simulink model "InteractiveArmModel_R2021a_v1"  (R2021a)
settings: Solver=ode4  StartTime=0.0  StopTime=3000  FixedStep=1/150  MaxStep=1/50  MinStep=1/200  RelTol=1e-5  AbsTol=1e-6  EnableMultiTasking=on
model workspace (MAT data in the model file):
  MaxEccentricFlexor = 0.5
  PoleZ = 0.85
  SampleTime = 0.05
  musNoise = 0
  musNoiseLevel = Simulink.Parameter
  musNoiseLevel.Value = 15.23
  musNoiseLevel.DataType = 'auto'
  musNoiseLevel.Dimensions = [1 1]
libraries: simulink x1
(part 1 of 3)
Description:
  | An interactive musculoskeletal model controllable with electromyography.
settings Model: SILPILModeSetting=veronly  PacingRate=1000  ExtModeTrigDuration=2  VariantFading=off  OrderedModelArguments=off  Creator=Christopher J. Hasson  LastModifiedBy=cjhas
settings SolverCC: AutoScaleAbsTol=off  InitialStep=1/10  ZeroCrossAlgorithm=Adaptive  AlgebraicLoopSolver=TrustRegion
settings OptimizationCC: DefaultParameterBehavior=Inlined  EnhancedBackFolding=on  PassReuseOutputArgsAs=Individual arguments  ZeroExternalMemoryAtStartup=off  ZeroInternalMemoryAtStartup=off  MaxStackSize=64  OptimizeBlockOrder=speed  DifferentSizesBufferReuse=on  OptimizationCustomize=off  EfficientTunableParamExpr=on
settings DebuggingCC: ReadBeforeWriteMsg=DisableAll  WriteAfterWriteMsg=DisableAll  WriteAfterReadMsg=DisableAll  MultiTaskDSMMsg=none  ParameterTunabilityLossMsg=error  SFMachineParentedDataDiag=warning
settings HardwareCC: ProdBitPerInt=16  ProdBitPerPointer=16  ProdBitPerSizeT=16  ProdBitPerPtrDiffT=16  ProdLargestAtomicFloat=None  ProdWordSize=8  ProdHWDeviceType=Atmel->AVR  UseEmbeddedCoderFeatures=off
settings ModelReferenceCC: UpdateModelReferenceTargets=IfOutOfDate
settings SFSimCC: SFSimEcho=off  MATLABDynamicMemAlloc=off
settings RTWCC: SystemTargetFile=ert.tlc  TemplateMakefile=ert_default_tmf  Toolchain=Arduino AVR  BuildConfiguration=Faster Runs
settings CodeAppCC: ForceParamTrailComments=on  IgnoreCustomStorageClasses=off  OperatorAnnotations=on  SimulinkDataObjDesc=on  SFDataObjDesc=on  InsertBlockDesc=on
settings ERTTargetCC: SupportContinuousTime=on  SupportNonInlinedSFcns=on  SupportVariableSizeSignals=on  ExtModeStaticAllocSize=250  ERTCustomFileTemplate=example_file_process.tlc

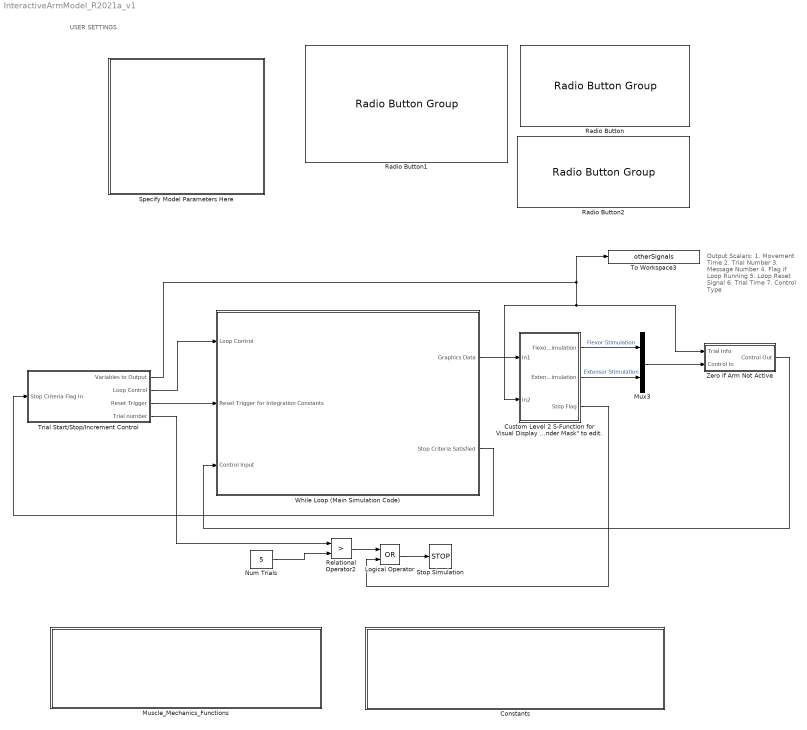
== system InteractiveArmModel_R2021a_v1 ==
  note: Output Scalars:
      | 1. Movement Time
      | 2. Trial Number
      | 3. Message Number
      | 4. Flag if Loop Running
      | 5. Loop Reset Signal
      | 6. Trial Time
      | 7. Control Type
  note: USER SETTINGS
  Constants : Subsystem
  "Custom Level 2 S-Function for Visual Display and Controls [Calls \"InteractiveDisplay.m\"] Select \"Look Under Mask\" to edit." : Subsystem  mask(Mutiple XY Graph){number_of_trajectories=2, axis_limits=[-0.5 0.5 -0.5 0.5], sample_time=0.01}
      mask prompts: number_of_trajectories "Number of Trajectories"; axis_limits "Axis Limits"; sample_time "Sample Time"
      mask Display: plot([.05 .95 .95 .05 .05],[.45 .45 .95 .95 .45], 0.5+cos(0:0.1:2*pi)*0.3,0.7+sin(0:0.1:2*pi)*0.2)
  Logical Operator : Logic  Operator=OR  AllPortsSameDT=off  OutDataTypeStr=boolean
  Muscle_Mechanics_Functions : Subsystem
  Mux3 : Mux  Inputs=2
  Num Trials : Constant  Value=5
  Radio Button : RadioButtonGroup  LabelPosition=Hide  SelectedLabel=Keyboard  ButtonGroupName=Control Mode
      settings: Values={{'Keyboard', 'Mouse', 'EMG'}, [0 1 2]}
  Radio Button1 : RadioButtonGroup  LabelPosition=Hide  SelectedLabel=Muscle Model  ButtonGroupName=Actuation
      settings: Values={{'Muscle Model', 'Force Generator', 'Torque Generator'}, [0 1 2]}
  Radio Button2 : RadioButtonGroup  LabelPosition=Hide  SelectedLabel=Normal  ButtonGroupName=Model Muscle Strength
      settings: Values={{'Normal', 'Weak (50% Reduction)'}, [0 1]}
  Relational Operator2 : RelationalOperator  Operator=>  RndMeth=Simplest
  Specify Model Parameters Here : Subsystem
  Stop Simulation : Stop
  To Workspace3 : ToWorkspace  VariableName=otherSignals  SaveFormat=Timeseries  SampleTime=-1
  Trial Start/Stop/Increment Control : Subsystem
  While Loop (Main Simulation Code) : Subsystem  TreatAsAtomicUnit=on
  Zero if Arm Not Active : Subsystem
  wires:
  While Loop (Main Simulation Code)/1(Graphics Data) -> "Custom Level 2 S-Function for Visual Display and Controls [Calls \"InteractiveDisplay.m\"] Select \"Look Under Mask\" to edit."/1(In1)
  Mux3/1 -> Zero if Arm Not Active/2(Control In)
  Zero if Arm Not Active/1(Control Out) -> While Loop (Main Simulation Code)/3(Control Input)
  "Custom Level 2 S-Function for Visual Display and Controls [Calls \"InteractiveDisplay.m\"] Select \"Look Under Mask\" to edit."/1(Flexor Stimulation) -> Mux3/1  "Flexor Stimulation"
  "Custom Level 2 S-Function for Visual Display and Controls [Calls \"InteractiveDisplay.m\"] Select \"Look Under Mask\" to edit."/2(Extensor Stimulation) -> Mux3/2  "Extensor Stimulation"
  Num Trials/1 -> Relational Operator2/2
  Relational Operator2/1 -> Logical Operator/1
  "Custom Level 2 S-Function for Visual Display and Controls [Calls \"InteractiveDisplay.m\"] Select \"Look Under Mask\" to edit."/3(Stop Flag) -> Logical Operator/2
  Logical Operator/1 -> Stop Simulation/1
  Trial Start/Stop/Increment Control/1(Variables to Output) -> Zero if Arm Not Active/1(Trial Info), "Custom Level 2 S-Function for Visual Display and Controls [Calls \"InteractiveDisplay.m\"] Select \"Look Under Mask\" to edit."/2(In2), To Workspace3/1
  While Loop (Main Simulation Code)/2(Stop Criteria Satisfied) -> Trial Start/Stop/Increment Control/1(Stop Criteria Flag In)
  Trial Start/Stop/Increment Control/4(Trial number) -> Relational Operator2/1
  Trial Start/Stop/Increment Control/2(Loop Control) -> While Loop (Main Simulation Code)/1(Loop Control)
  Trial Start/Stop/Increment Control/3(Reset Trigger) -> While Loop (Main Simulation Code)/2(Reset Trigger for Integration Constants)

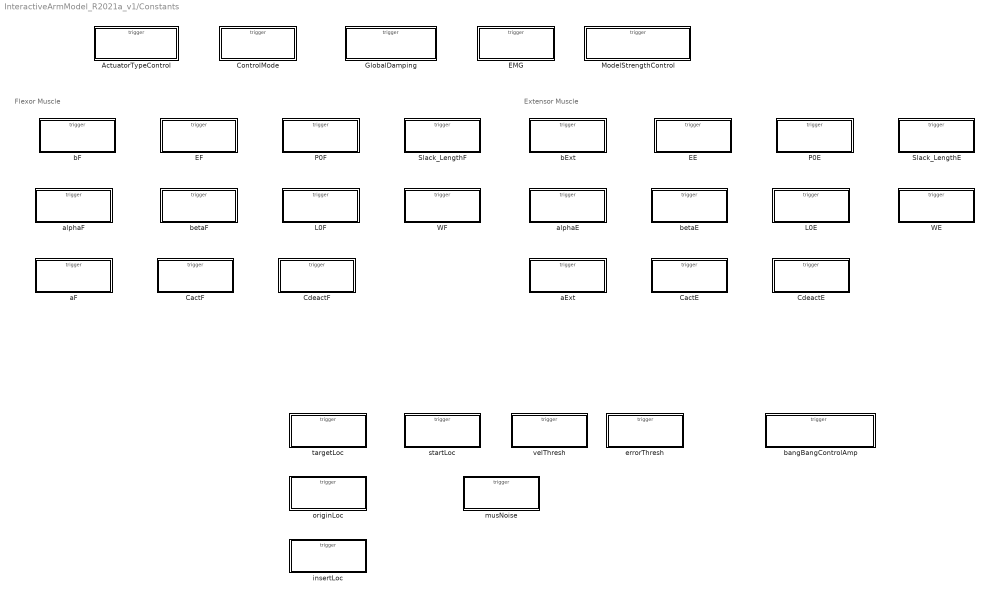
== system InteractiveArmModel_R2021a_v1/Constants ==
  note: Extensor Muscle
  note: Flexor Muscle
  ActuatorTypeControl : Subsystem  TreatAsAtomicUnit=on
  CactE : Subsystem  TreatAsAtomicUnit=on
  CactF : Subsystem  TreatAsAtomicUnit=on
  CdeactE : Subsystem  TreatAsAtomicUnit=on
  CdeactF : Subsystem  TreatAsAtomicUnit=on
  ControlMode : Subsystem  TreatAsAtomicUnit=on
  EE : Subsystem  TreatAsAtomicUnit=on
  EF : Subsystem  TreatAsAtomicUnit=on
  EMG : Subsystem  TreatAsAtomicUnit=on
  GlobalDamping : Subsystem  TreatAsAtomicUnit=on
  L0E : Subsystem  TreatAsAtomicUnit=on
  L0F : Subsystem  TreatAsAtomicUnit=on
  ModelStrengthControl : Subsystem  TreatAsAtomicUnit=on
  P0E : Subsystem  TreatAsAtomicUnit=on
  P0F : Subsystem  TreatAsAtomicUnit=on
  Slack_LengthE : Subsystem  TreatAsAtomicUnit=on
  Slack_LengthF : Subsystem  TreatAsAtomicUnit=on
  WE : Subsystem  TreatAsAtomicUnit=on
  WF : Subsystem  TreatAsAtomicUnit=on
  aExt : Subsystem  TreatAsAtomicUnit=on
  aF : Subsystem  TreatAsAtomicUnit=on
  alphaE : Subsystem  TreatAsAtomicUnit=on
  alphaF : Subsystem  TreatAsAtomicUnit=on
  bExt : Subsystem  TreatAsAtomicUnit=on
  bF : Subsystem  TreatAsAtomicUnit=on
  bangBangControlAmp : Subsystem  TreatAsAtomicUnit=on
  betaE : Subsystem  TreatAsAtomicUnit=on
  betaF : Subsystem  TreatAsAtomicUnit=on
  errorThresh : Subsystem  TreatAsAtomicUnit=on
  insertLoc : Subsystem  TreatAsAtomicUnit=on
  musNoise : Subsystem  TreatAsAtomicUnit=on
  originLoc : Subsystem  TreatAsAtomicUnit=on
  startLoc : Subsystem  TreatAsAtomicUnit=on
  targetLoc : Subsystem  TreatAsAtomicUnit=on
  velThresh : Subsystem  TreatAsAtomicUnit=on

== system InteractiveArmModel_R2021a_v1/Custom Level 2 S-Function for Visual Display and Controls [Calls "InteractiveDisplay.m"] Select "Look Under Mask" to edit. ==
  In1 : Inport
  In2 : Inport  Port=2
  Demux : Demux  Outputs=25
  Level-2 MATLAB S-Function : M-S-Function  FunctionName=InteractiveDisplay  Parameters=number_of_trajectories,axis_limits
  Flexor Stimulation : Outport
  Extensor Stimulation : Outport  Port=2
  Stop Flag : Outport  Port=3
  wires:
  Level-2 MATLAB S-Function/1 -> Demux/1
  Demux/1 -> Flexor Stimulation/1
  Demux/2 -> Extensor Stimulation/1
  In1/1 -> Level-2 MATLAB S-Function/1
  In2/1 -> Level-2 MATLAB S-Function/2
  Demux/3 -> Stop Flag/1

== system InteractiveArmModel_R2021a_v1/Muscle_Mechanics_Functions ==
  Contractile Element Excitation-Activation Relation : Subsystem  TreatAsAtomicUnit=on
  Contractile Element Force-Length Relation : Subsystem  TreatAsAtomicUnit=on
  Contractile Element Force-Velocity Relation : Subsystem  TreatAsAtomicUnit=on
  "Series-Elastic Element Stiffness Relation " : Subsystem  TreatAsAtomicUnit=on

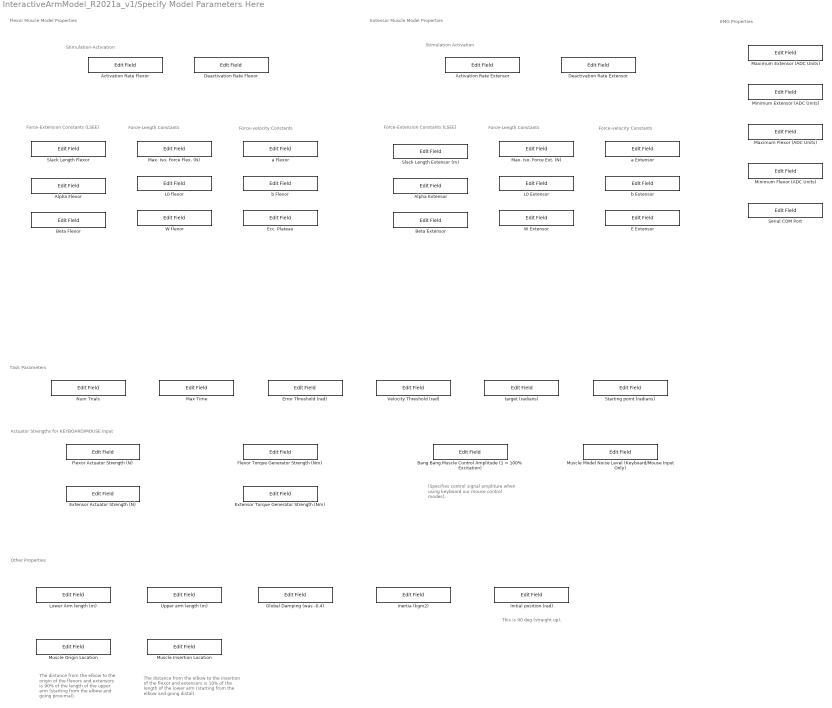
== system InteractiveArmModel_R2021a_v1/Specify Model Parameters Here ==
  note: (Specifies control signal ampliture when using keyboard our mouse control modes).
  note: EMG Properties
  note: Task Parameters
  note: Stimulation Activation
  note: Stimulation-Activation
  note: Force-velocity Constants
  note: Force-Extension Constants
      |  (LSEE)
  note: Force-Length Constants
  note: Flexor Muscle Model Properties
  note: Extensor Muscle Model Properties
  note: Force-velocity Constants
  note: Force-Extension Constants
      |  (LSEE)
  note: Force-Length Constants
  note: Actuator Strengths for KEYBOARD/MOUSE Input
  note: The distance from the elbow to the origin of the flexors and extensors is 90% of the length of the upper arm (starting from the elbow and going proximal).
  note: The distance from the elbow to the insertion of the flexor and extensors is 10% of the length of the lower arm (starting from the elbow and going distal).
  note: This is 90 deg (straight up).
  note: Other Properties
  Activation Rate Extensor : EditField  LabelPosition=Hide  ShowInitialText=on  Alignment=Center
  Activation Rate Flexor : EditField  LabelPosition=Hide  ShowInitialText=on  Alignment=Center
  Alpha Extensor : EditField  LabelPosition=Hide  ShowInitialText=on  Alignment=Center
  Alpha Flexor : EditField  LabelPosition=Hide  ShowInitialText=on  Alignment=Center
  Bang Bang Muscle Control Amplitude (1 = 100% Excitation) : EditField  LabelPosition=Hide  ShowInitialText=on  Alignment=Center
  Beta Extensor : EditField  LabelPosition=Hide  ShowInitialText=on  Alignment=Center
  Beta Flexor : EditField  LabelPosition=Hide  ShowInitialText=on  Alignment=Center
  Deactivation Rate Extensor : EditField  LabelPosition=Hide  ShowInitialText=on  Alignment=Center
  Deactivation Rate Flexor : EditField  LabelPosition=Hide  ShowInitialText=on  Alignment=Center
  E Extensor : EditField  LabelPosition=Hide  ShowInitialText=on  Alignment=Center
  Ecc. Plateau : EditField  LabelPosition=Hide  ShowInitialText=on  Alignment=Center
  Error Threshold (rad) : EditField  LabelPosition=Hide  ShowInitialText=on  Alignment=Center
  Extensor Actuator Strength (N) : EditField  LabelPosition=Hide  ShowInitialText=on  Alignment=Center
  Extensor Torque Generator Strength (Nm) : EditField  LabelPosition=Hide  ShowInitialText=on  Alignment=Center
  Flexor Actuator Strength (N) : EditField  LabelPosition=Hide  ShowInitialText=on  Alignment=Center
  Flexor Torque Generator Strength (Nm) : EditField  LabelPosition=Hide  ShowInitialText=on  Alignment=Center
  Global Damping (was -0.4) : EditField  LabelPosition=Hide  ShowInitialText=on  Alignment=Center
  Inertia (kgm2) : EditField  LabelPosition=Hide  ShowInitialText=on  Alignment=Center
  Initial position (rad) : EditField  LabelPosition=Hide  ShowInitialText=on  Alignment=Center
  L0 Extensor : EditField  LabelPosition=Hide  ShowInitialText=on  Alignment=Center
  L0 flexor : EditField  LabelPosition=Hide  ShowInitialText=on  Alignment=Center
  Lower Arm length (m) : EditField  LabelPosition=Hide  ShowInitialText=on  Alignment=Center
  Max Time : EditField  LabelPosition=Hide  ShowInitialText=on  Alignment=Center
  Max. Iso. Force Ext. (N) : EditField  LabelPosition=Hide  ShowInitialText=on  Alignment=Center
  Max. Iso. Force Flex. (N) : EditField  LabelPosition=Hide  ShowInitialText=on  Alignment=Center
  Maximum Extensor (ADC Units) : EditField  LabelPosition=Hide  ShowInitialText=on  Alignment=Center
  Maximum Flexor (ADC Units) : EditField  LabelPosition=Hide  ShowInitialText=on  Alignment=Center
  Minimum Extensor (ADC Units) : EditField  LabelPosition=Hide  ShowInitialText=on  Alignment=Center
  Minimum Flexor (ADC Units) : EditField  LabelPosition=Hide  ShowInitialText=on  Alignment=Center
  Muscle Insertion Location : EditField  LabelPosition=Hide  ShowInitialText=on  Alignment=Center
  Muscle Model Noise Level (Keyboard/Mouse Input Only) : EditField  LabelPosition=Hide  ShowInitialText=on  Alignment=Center
  Muscle Origin Location : EditField  LabelPosition=Hide  ShowInitialText=on  Alignment=Center
  Num Trials : EditField  LabelPosition=Hide  ShowInitialText=on  Alignment=Center
  Serial COM Port : EditField  LabelPosition=Hide  ShowInitialText=on  Alignment=Center
  Slack Length Extensor (m) : EditField  LabelPosition=Hide  ShowInitialText=on  Alignment=Center
  Slack Length Flexor : EditField  LabelPosition=Hide  ShowInitialText=on  Alignment=Center
  Starting point (radians) : EditField  LabelPosition=Hide  ShowInitialText=on  Alignment=Center
  Upper arm length (m) : EditField  LabelPosition=Hide  ShowInitialText=on  Alignment=Center
  Velocity Threshold (rad) : EditField  LabelPosition=Hide  ShowInitialText=on  Alignment=Center
  W Extensor : EditField  LabelPosition=Hide  ShowInitialText=on  Alignment=Center
  W flexor : EditField  LabelPosition=Hide  ShowInitialText=on  Alignment=Center
  a Extensor : EditField  LabelPosition=Hide  ShowInitialText=on  Alignment=Center
  a Flexor : EditField  LabelPosition=Hide  ShowInitialText=on  Alignment=Center
  b Extensor : EditField  LabelPosition=Hide  ShowInitialText=on  Alignment=Center
  b Flexor : EditField  LabelPosition=Hide  ShowInitialText=on  Alignment=Center
  target (radians) : EditField  LabelPosition=Hide  ShowInitialText=on  Alignment=Center

== system InteractiveArmModel_R2021a_v1/Trial Start//Stop//Increment Control ==
  note: 1 = Trial is active (Stop critiera not satisfied and trial time hasn't reached limit).
  Stop Criteria Flag In : Inport
  Counter for Trial Number : Subsystem  TreatAsAtomicUnit=on
  Data Type Conversion2 : DataTypeConversion
  Delay : Delay  DelayLength=50  InitialCondition=0
  Extract Movement Time : Subsystem  TreatAsAtomicUnit=on
  Flag for What Phase Trial is In : Subsystem
  Function Caller : FunctionCaller  FunctionPrototype=y = Constants.ControlMode()  OutputArgumentSpecifications=<Enter example>
  Mux : Mux  Inputs=7
  Reset Trigger Logic : Subsystem
  Stop Criteria Flag Control (Between Trials) : Subsystem
  Subsystem : Subsystem
  Subsystem1 : Subsystem
  Subsystem2 : Subsystem
  Variables to Output : Outport
  Loop Control : Outport  Port=2
  Reset Trigger : Outport  Port=3
  Trial number : Outport  Port=4
  wires:
  Subsystem2/1(IC) -> Loop Control/1, Extract Movement Time/Trigger, Mux/4
  Reset Trigger Logic/1(Reset Trigger) -> Reset Trigger/1, Data Type Conversion2/1
  Subsystem/1(Simulation Time) -> Subsystem2/1(Simulation Time)
  Subsystem1/2(Trial Time Flag) -> Flag for What Phase Trial is In/1(Trial Time Flag)
  Mux/1 -> Variables to Output/1
  Stop Criteria Flag Control (Between Trials)/1(Stop Criteria Flag Out) -> Subsystem1/2(Stop Criteria Flag), Flag for What Phase Trial is In/2(Stop Criteria Flag), Reset Trigger Logic/2(Stop Criteria Flag)
  Flag for What Phase Trial is In/1(message display) -> Mux/3
  Counter for Trial Number/1(Trial Number Switch) -> Trial number/1, Mux/2  "Trial number"
  Extract Movement Time/1(Movement Time) -> Mux/1
  Data Type Conversion2/1 -> Mux/5  "Reset"
  Subsystem/2(Trial Time) -> Counter for Trial Number/Trigger, Extract Movement Time/1(Trial Time), Mux/6, Reset Trigger Logic/1(Trial Time), Subsystem1/1(Trial Time)
  Function Caller/1 -> Mux/7
  Delay/1 -> Subsystem/1(In1)
  Subsystem1/1(StopCriteria&TrialTime Flag) -> Subsystem2/2(StopCriteria&TrialTime Flag), Delay/1
  Stop Criteria Flag In/1 -> Stop Criteria Flag Control (Between Trials)/1(Stop Criteria Flag In)

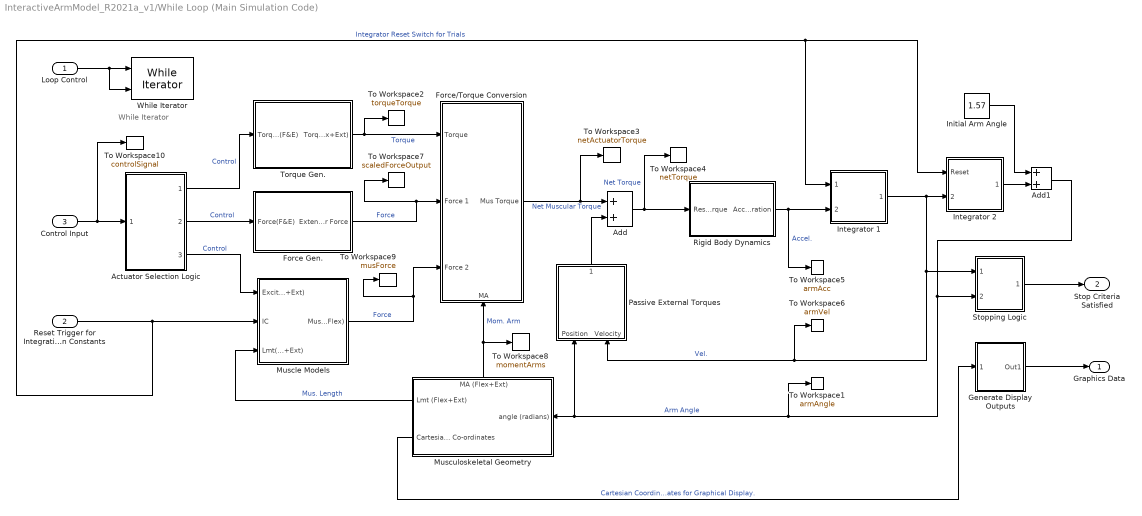
== system InteractiveArmModel_R2021a_v1/While Loop (Main Simulation Code) ==
  note: While Iterator
  Loop Control : Inport
  Reset Trigger for Integration Constants : Inport  Port=2
  Control Input : Inport  Port=3
  Actuator Selection Logic : Subsystem
  Add : Sum
  Add1 : Sum
  Force Gen. : Subsystem
  Force/Torque Conversion : Subsystem
      settings: PortSchema="{\"entries\":[{\"content\":{\"sides\":[{\"content\":{\"connectorIds\":[\"In1\",\"In2\",\"In3\"]},\"type\":\"ConnectorPlacement.EquallySpacedRectSide\",\"uuid\":\"3849f213-61a2-4952-aa4f-2be59b7e729a\"},{\"content\":{\"connectorIds\":[\"Out1\"],\"side\":\"RIGHT\"},\"type\":\"ConnectorPlacement.EquallySpacedRectSide\",\"uuid\":\"a03946d5-4adf-48f1-b5d4-befc99ec4479\"},{\"content\":{\"connectorIds\":[],\"side\":\"TOP\"},\"type\":\"ConnectorPlacement.EquallySpacedRectSide\",\"uuid\":\"26cd925e-d209-4c63-b11b-6b56fbf295e7\"},{\"content\":{\"connectorIds\":[\"In4\"],\"side\":\"BOTTOM\"},\"type\":\"ConnectorPlacement.EquallySpacedRectSide\",\"uuid\":\"3307b9fa-59bc-4d23-82dd-e0fccabeb078\"}]},\"type\":\"ConnectorPlacement.EquallySpacedConnector\",\"uuid\":\"629632a8-6ad9-402b-9008-6a2bdbad6252\"}],\"packageUris\":[\"http://schema.mathworks.com/mf0/Connector/R2020b\"],\"version\":\"1.0\"}"
  Generate Display Outputs : Subsystem
      settings: PortSchema="{\"entries\":[{\"content\":{\"sides\":[{\"content\":{\"connectorIds\":[\"Out1\"]},\"type\":\"ConnectorPlacement.EquallySpacedRectSide\",\"uuid\":\"907c53ba-e25a-48a3-8580-f053d35e8a8b\"},{\"content\":{\"connectorIds\":[\"In1\"],\"side\":\"RIGHT\"},\"type\":\"ConnectorPlacement.EquallySpacedRectSide\",\"uuid\":\"e6d73d20-9b05-462a-b014-b0e267ff725b\"},{\"content\":{\"connectorIds\":[],\"side\":\"TOP\"},\"type\":\"ConnectorPlacement.EquallySpacedRectSide\",\"uuid\":\"2f7da445-9925-4d1a-82a6-929fe983f70f\"},{\"content\":{\"connectorIds\":[],\"side\":\"BOTTOM\"},\"type\":\"ConnectorPlacement.EquallySpacedRectSide\",\"uuid\":\"a6d810bc-350c-475e-931f-1209d385d960\"}]},\"type\":\"ConnectorPlacement.EquallySpacedConnector\",\"uuid\":\"aaa2837d-0021-4fae-b2fd-c5fc5dc28df7\"}],\"packageUris\":[\"http://schema.mathworks.com/mf0/Connector/R2020b\"],\"version\":\"1.0\"}"
  Initial Arm Angle : Constant  Value=1.57
  Integrator 1 : Subsystem
  Integrator 2 : Subsystem
  Muscle Models : Subsystem
  Musculoskeletal Geometry : Subsystem
      settings: PortSchema="{\"entries\":[{\"content\":{\"sides\":[{\"content\":{\"connectorIds\":[]},\"type\":\"ConnectorPlacement.EquallySpacedRectSide\",\"uuid\":\"8c940fc8-64df-4196-ac14-c49096b27983\"},{\"content\":{\"connectorIds\":[\"Out1\"],\"side\":\"RIGHT\"},\"type\":\"ConnectorPlacement.EquallySpacedRectSide\",\"uuid\":\"009c2c09-14e0-422f-89fa-0830fe563124\"},{\"content\":{\"connectorIds\":[\"Out2\",\"Out3\"],\"side\":\"TOP\"},\"type\":\"ConnectorPlacement.EquallySpacedRectSide\",\"uuid\":\"84c5c2e7-ffda-4103-9912-3de94ad78eb8\"},{\"content\":{\"connectorIds\":[\"In1\"],\"side\":\"BOTTOM\"},\"type\":\"ConnectorPlacement.EquallySpacedRectSide\",\"uuid\":\"bc27ef22-e0e2-497d-b784-b185d27dfcbe\"}]},\"type\":\"ConnectorPlacement.EquallySpacedConnector\",\"uuid\":\"d3fcff10-aff8-4015-b565-4cd041df8c8d\"}],\"packageUris\":[\"http://schema.mathworks.com/mf0/Connector/19700101\"],\"version\":\"1.0\"}"
  Passive External Torques : Subsystem
      settings: PortSchema="{\"entries\":[{\"content\":{\"sides\":[{\"content\":{\"connectorIds\":[]},\"type\":\"ConnectorPlacement.EquallySpacedRectSide\",\"uuid\":\"d0cf707c-0e80-49c4-a718-ce527ee82e97\"},{\"content\":{\"connectorIds\":[],\"side\":\"RIGHT\"},\"type\":\"ConnectorPlacement.EquallySpacedRectSide\",\"uuid\":\"ee5fdd45-e6b2-4d3c-954e-bdf912ed2468\"},{\"content\":{\"connectorIds\":[\"Out1\"],\"side\":\"TOP\"},\"type\":\"ConnectorPlacement.EquallySpacedRectSide\",\"uuid\":\"54b9e406-3152-4f28-af7f-87d9f53bbd53\"},{\"content\":{\"connectorIds\":[\"In1\",\"In2\"],\"side\":\"BOTTOM\"},\"type\":\"ConnectorPlacement.EquallySpacedRectSide\",\"uuid\":\"aacaddaa-a99e-4423-a15d-1a454195a54f\"}]},\"type\":\"ConnectorPlacement.EquallySpacedConnector\",\"uuid\":\"bf7677b5-f77f-4845-ae2c-48e3ea7a2b50\"}],\"packageUris\":[\"http://schema.mathworks.com/mf0/Connector/19700101\"],\"version\":\"1.0\"}"
  Rigid Body Dynamics : Subsystem
  Stopping Logic : Subsystem
  To Workspace1 : ToWorkspace  VariableName=armAngle  SaveFormat=Timeseries  SampleTime=-1
  To Workspace10 : ToWorkspace  VariableName=controlSignal  SaveFormat=Timeseries  SampleTime=-1
  To Workspace2 : ToWorkspace  VariableName=torqueTorque  SaveFormat=Timeseries  SampleTime=-1
  To Workspace3 : ToWorkspace  VariableName=netActuatorTorque  SaveFormat=Timeseries  SampleTime=-1
  To Workspace4 : ToWorkspace  VariableName=netTorque  SaveFormat=Timeseries  SampleTime=-1
  To Workspace5 : ToWorkspace  VariableName=armAcc  SaveFormat=Timeseries  SampleTime=-1
  To Workspace6 : ToWorkspace  VariableName=armVel  SaveFormat=Timeseries  SampleTime=-1
  To Workspace7 : ToWorkspace  VariableName=scaledForceOutput  SampleTime=-1
  To Workspace8 : ToWorkspace  VariableName=momentArms  SaveFormat=Timeseries  SampleTime=-1
  To Workspace9 : ToWorkspace  VariableName=musForce  SampleTime=-1
  Torque Gen. : Subsystem
  While Iterator : WhileIterator  MaxIters=1  OutputDataType=double
  Graphics Data : Outport
  Stop Criteria Satisfied : Outport  Port=2
  wires:
  Loop Control/1 -> While Iterator/2, While Iterator/1
  Force/Torque Conversion/1(Mus Torque) -> To Workspace3/1, Add/1  "Net Muscular Torque"
  Passive External Torques/1(Net External Torque) -> Add/2
  Add/1 -> To Workspace4/1, Rigid Body Dynamics/1(Resultant torque)  "Net Torque"
  Muscle Models/1(Muscle Force (Ext+Flex)) -> To Workspace9/1, Force/Torque Conversion/3(Force 2)  "Force"
  Force Gen./1(Extensor Force) -> To Workspace7/1, Force/Torque Conversion/2(Force 1)  "Force"
  Musculoskeletal Geometry/1(MA (Flex+Ext)) -> Force/Torque Conversion/4(MA), To Workspace8/1  "Mom. Arm"
  Musculoskeletal Geometry/2(Cartesian Co-ordinates) -> Generate Display Outputs/1(Cartesian Co-ordinates)  "Cartesian Coordinates for Graphical Display."
  Add1/1 -> To Workspace1/1, Musculoskeletal Geometry/1(angle (radians)), Passive External Torques/1(Position), Stopping Logic/2(Angle (radians))  "Arm Angle"
  Musculoskeletal Geometry/3(Lmt (Flex+Ext)) -> Muscle Models/3(Lmt(flex+Ext))  "Mus. Length"
  Torque Gen./1(Torque (flex+Ext)) -> To Workspace2/1, Force/Torque Conversion/1(Torque)  "Torque"
  Generate Display Outputs/1(Out1) -> Graphics Data/1
  Reset Trigger for Integration Constants/1 -> Muscle Models/2(IC), Integrator 2/1(Reset), Integrator 1/1(Reset1)  "Integrator Reset Switch for Trials"
  Rigid Body Dynamics/1(" Acceleration") -> Integrator 1/2(Arm Accel.), To Workspace5/1  "Accel."
  Stopping Logic/1(Out2) -> Stop Criteria Satisfied/1
  Control Input/1 -> To Workspace10/1, Actuator Selection Logic/1(Control Input)
  Actuator Selection Logic/1(Torque Control Signal) -> Torque Gen./1(Torque(F&E))  "Control"
  Actuator Selection Logic/2(Force Actuator Control Signal) -> Force Gen./1(Force(F&E))  "Control"
  Integrator 1/1(Arm Vel.) -> To Workspace6/1, Passive External Torques/2(Velocity), Stopping Logic/1(Velocity (rad/s)), Integrator 2/2(Arm Vel.)  "Vel."
  Integrator 2/1(PosOut) -> Add1/2
  Initial Arm Angle/1 -> Add1/1
  Actuator Selection Logic/3(MuscleControlSignal) -> Muscle Models/1(Excitation(flex+Ext))  "Control"

== system InteractiveArmModel_R2021a_v1/Zero if Arm Not Active ==
  Trial Info : Inport
  Control In : Inport  Port=2
  Constant1 : Constant  Value=0
  Constant3 : Constant  Value=0
  Demux : Demux  Outputs=2
  Demux1 : Demux  Outputs=7
  If Action Subsystem1 : Subsystem  TreatAsAtomicUnit=on
  If Action Subsystem10 : Subsystem  TreatAsAtomicUnit=on
  If Action Subsystem11 : Subsystem  TreatAsAtomicUnit=on
  If Action Subsystem2 : Subsystem  TreatAsAtomicUnit=on
  If1 : If  IfExpression=u1 == 0
  If5 : If  IfExpression=u1 == 0
  Logical Operator : Logic  AllPortsSameDT=off  OutDataTypeStr=boolean
  Merge1 : Merge
  Merge4 : Merge
  Mux : Mux  Inputs=2
  Control Out : Outport
  wires:
  Constant3/1 -> If Action Subsystem10/1(In1)
  If Action Subsystem10/1(Out1) -> Merge4/1
  If5/1 -> If Action Subsystem10/Action
  If5/2 -> If Action Subsystem11/Action
  Merge4/1 -> Mux/1
  Mux/1 -> Control Out/1
  If Action Subsystem11/1(Out1) -> Merge4/2
  Constant1/1 -> If Action Subsystem1/1(In1)
  If1/1 -> If Action Subsystem1/Action
  Control In/1 -> Demux/1
  Demux/1 -> If Action Subsystem11/1(" ")  "Flexor"
  If1/2 -> If Action Subsystem2/Action
  Demux/2 -> If Action Subsystem2/1(" ")  "Extensor"
  If Action Subsystem2/1(Out1) -> Merge1/2
  If Action Subsystem1/1(Out1) -> Merge1/1
  Merge1/1 -> Mux/2
  Trial Info/1 -> Demux1/1
  Demux1/4 -> Logical Operator/1  "IC"
  Demux1/5 -> Logical Operator/2  "Reset"
  Logical Operator/1 -> If1/1, If5/1

== system InteractiveArmModel_R2021a_v1/Constants/ActuatorTypeControl ==
  ActuatorType : TriggerPort  TriggerType=function-call  IsSimulinkFunction=on  FunctionName=ActuatorType  FunctionVisibility=scoped  VariantControl=(inherit)
  Constant10 : Constant  Value=0
  y : ArgOut  DisableCoverage=on  ArgumentName=y
  wires:
  Constant10/1 -> y/1

== system InteractiveArmModel_R2021a_v1/Constants/CactE ==
  CactE : TriggerPort  TriggerType=function-call  IsSimulinkFunction=on  FunctionName=CactE  FunctionVisibility=scoped  VariantControl=(inherit)
  Flex Act Constant : Constant  Value=0.03
  y : ArgOut  DisableCoverage=on  ArgumentName=y
  wires:
  Flex Act Constant/1 -> y/1

== system InteractiveArmModel_R2021a_v1/Constants/CactF ==
  CactF : TriggerPort  TriggerType=function-call  IsSimulinkFunction=on  FunctionName=CactF  FunctionVisibility=scoped  VariantControl=(inherit)
  Flex Act Constant : Constant  Value=0.03
  y : ArgOut  DisableCoverage=on  ArgumentName=y
  wires:
  Flex Act Constant/1 -> y/1

== system InteractiveArmModel_R2021a_v1/Constants/CdeactE ==
  CdeactE : TriggerPort  TriggerType=function-call  IsSimulinkFunction=on  FunctionName=CdeactE  FunctionVisibility=scoped  VariantControl=(inherit)
  Ext Act Constant : Constant  Value=0.06
  y : ArgOut  DisableCoverage=on  ArgumentName=y
  wires:
  Ext Act Constant/1 -> y/1

== system InteractiveArmModel_R2021a_v1/Constants/CdeactF ==
  CdeactF : TriggerPort  TriggerType=function-call  IsSimulinkFunction=on  FunctionName=CdeactF  FunctionVisibility=scoped  VariantControl=(inherit)
  Flex Deact Constant : Constant  Value=0.06
  y : ArgOut  DisableCoverage=on  ArgumentName=y
  wires:
  Flex Deact Constant/1 -> y/1

== system InteractiveArmModel_R2021a_v1/Constants/ControlMode ==
  ControlMode : TriggerPort  TriggerType=function-call  IsSimulinkFunction=on  FunctionName=ControlMode  FunctionVisibility=scoped  VariantControl=(inherit)
  ControlModeConstant : Constant  Value=0
  y : ArgOut  DisableCoverage=on  ArgumentName=y
  wires:
  ControlModeConstant/1 -> y/1

== system InteractiveArmModel_R2021a_v1/Constants/EE ==
  EE : TriggerPort  TriggerType=function-call  IsSimulinkFunction=on  FunctionName=EE  FunctionVisibility=scoped  VariantControl=(inherit)
  eccentricExtensor : Constant  Value=3
  y : ArgOut  DisableCoverage=on  ArgumentName=y
  wires:
  eccentricExtensor/1 -> y/1

== system InteractiveArmModel_R2021a_v1/Constants/EF ==
  EF : TriggerPort  TriggerType=function-call  IsSimulinkFunction=on  FunctionName=EF  FunctionVisibility=scoped  VariantControl=(inherit)
  eccentricFlexor : Constant  Value=2.58
  y : ArgOut  DisableCoverage=on  ArgumentName=y
  wires:
  eccentricFlexor/1 -> y/1

== system InteractiveArmModel_R2021a_v1/Constants/EMG ==
  EMG : TriggerPort  TriggerType=function-call  IsSimulinkFunction=on  FunctionName=EMG  FunctionVisibility=scoped  VariantControl=(inherit)
  "EMG vs Button " : Constant  Value=0
  y : ArgOut  DisableCoverage=on  ArgumentName=y
  wires:
  "EMG vs Button "/1 -> y/1

== system InteractiveArmModel_R2021a_v1/Constants/GlobalDamping ==
  GlobalDamping : TriggerPort  TriggerType=function-call  IsSimulinkFunction=on  FunctionName=GlobalDamping  FunctionVisibility=scoped  VariantControl=(inherit)
  GlobalDampingConstant : Constant  Value=0
  y : ArgOut  DisableCoverage=on  ArgumentName=y
  wires:
  GlobalDampingConstant/1 -> y/1

== system InteractiveArmModel_R2021a_v1/Constants/L0E ==
  L0E : TriggerPort  TriggerType=function-call  IsSimulinkFunction=on  FunctionName=L0E  FunctionVisibility=scoped  VariantControl=(inherit)
  optLenExtensor : Constant  Value=0.223
  y : ArgOut  DisableCoverage=on  ArgumentName=y
  wires:
  optLenExtensor/1 -> y/1

== system InteractiveArmModel_R2021a_v1/Constants/L0F ==
  L0F : TriggerPort  TriggerType=function-call  IsSimulinkFunction=on  FunctionName=L0F  FunctionVisibility=scoped  VariantControl=(inherit)
  optLenFlex : Constant  Value=0.223
  y : ArgOut  DisableCoverage=on  ArgumentName=y
  wires:
  optLenFlex/1 -> y/1

== system InteractiveArmModel_R2021a_v1/Constants/ModelStrengthControl ==
  ModelStrengthControl : TriggerPort  TriggerType=function-call  IsSimulinkFunction=on  FunctionName=ModelStrengthControl  FunctionVisibility=scoped  VariantControl=(inherit)
  ModelStrengthConstant : Constant  Value=0
  y : ArgOut  DisableCoverage=on  ArgumentName=y
  wires:
  ModelStrengthConstant/1 -> y/1

== system InteractiveArmModel_R2021a_v1/Constants/P0E ==
  P0E : TriggerPort  TriggerType=function-call  IsSimulinkFunction=on  FunctionName=P0E  FunctionVisibility=scoped  VariantControl=(inherit)
  MaxIsoExtensor : Constant  Value=1000
  y : ArgOut  DisableCoverage=on  ArgumentName=y
  wires:
  MaxIsoExtensor/1 -> y/1

== system InteractiveArmModel_R2021a_v1/Constants/P0F ==
  P0F : TriggerPort  TriggerType=function-call  IsSimulinkFunction=on  FunctionName=P0F  FunctionVisibility=scoped  VariantControl=(inherit)
  MaxIsoFlexor : Constant  Value=1000
  y : ArgOut  DisableCoverage=on  ArgumentName=y
  wires:
  MaxIsoFlexor/1 -> y/1

== system InteractiveArmModel_R2021a_v1/Constants/Slack_LengthE ==
  Slack_lengthE : TriggerPort  TriggerType=function-call  IsSimulinkFunction=on  FunctionName=Slack_lengthE  FunctionVisibility=scoped  VariantControl=(inherit)
  SlackLenExt : Constant  Value=0.11
  y : ArgOut  DisableCoverage=on  ArgumentName=y
  wires:
  SlackLenExt/1 -> y/1

== system InteractiveArmModel_R2021a_v1/Constants/Slack_LengthF ==
  Slack_lengthF : TriggerPort  TriggerType=function-call  IsSimulinkFunction=on  FunctionName=Slack_lengthF  FunctionVisibility=scoped  VariantControl=(inherit)
  Slack_Length_Flexor : Constant  Value=0.12
  y : ArgOut  DisableCoverage=on  ArgumentName=y
  wires:
  Slack_Length_Flexor/1 -> y/1

== system InteractiveArmModel_R2021a_v1/Constants/WE ==
  WE : TriggerPort  TriggerType=function-call  IsSimulinkFunction=on  FunctionName=WE  FunctionVisibility=scoped  VariantControl=(inherit)
  widthExtensor : Constant  Value=0.036
  y : ArgOut  DisableCoverage=on  ArgumentName=y
  wires:
  widthExtensor/1 -> y/1

== system InteractiveArmModel_R2021a_v1/Constants/WF ==
  WF : TriggerPort  TriggerType=function-call  IsSimulinkFunction=on  FunctionName=WF  FunctionVisibility=scoped  VariantControl=(inherit)
  widthFlexor : Constant  Value=0.036
  y : ArgOut  DisableCoverage=on  ArgumentName=y
  wires:
  widthFlexor/1 -> y/1

== system InteractiveArmModel_R2021a_v1/Constants/aExt ==
  aE : TriggerPort  TriggerType=function-call  IsSimulinkFunction=on  FunctionName=aE  FunctionVisibility=scoped  VariantControl=(inherit)
  hillAExtensor : Constant  Value=360
  y : ArgOut  DisableCoverage=on  ArgumentName=y
  wires:
  hillAExtensor/1 -> y/1

== system InteractiveArmModel_R2021a_v1/Constants/aF ==
  aF : TriggerPort  TriggerType=function-call  IsSimulinkFunction=on  FunctionName=aF  FunctionVisibility=scoped  VariantControl=(inherit)
  hillAFlexor : Constant  Value=360
  y : ArgOut  DisableCoverage=on  ArgumentName=y
  wires:
  hillAFlexor/1 -> y/1

== system InteractiveArmModel_R2021a_v1/Constants/alphaE ==
  alphaE : TriggerPort  TriggerType=function-call  IsSimulinkFunction=on  FunctionName=alphaE  FunctionVisibility=scoped  VariantControl=(inherit)
  alphaExtensor : Constant  Value=605
  y : ArgOut  DisableCoverage=on  ArgumentName=y
  wires:
  alphaExtensor/1 -> y/1

== system InteractiveArmModel_R2021a_v1/Constants/alphaF ==
  alphaF : TriggerPort  TriggerType=function-call  IsSimulinkFunction=on  FunctionName=alphaF  FunctionVisibility=scoped  VariantControl=(inherit)
  alphaFlexor : Constant  Value=605
  y : ArgOut  DisableCoverage=on  ArgumentName=y
  wires:
  alphaFlexor/1 -> y/1

== system InteractiveArmModel_R2021a_v1/Constants/bExt ==
  bE : TriggerPort  TriggerType=function-call  IsSimulinkFunction=on  FunctionName=bE  FunctionVisibility=scoped  VariantControl=(inherit)
  hillBExtensor : Constant  Value=0.28
  y : ArgOut  DisableCoverage=on  ArgumentName=y
  wires:
  hillBExtensor/1 -> y/1

== system InteractiveArmModel_R2021a_v1/Constants/bF ==
  bF : TriggerPort  TriggerType=function-call  IsSimulinkFunction=on  FunctionName=bF  FunctionVisibility=scoped  VariantControl=(inherit)
  hillBFlexor : Constant  Value=0.28
  y : ArgOut  DisableCoverage=on  ArgumentName=y
  wires:
  hillBFlexor/1 -> y/1

== system InteractiveArmModel_R2021a_v1/Constants/bangBangControlAmp ==
  bangBangControlAmp : TriggerPort  TriggerType=function-call  IsSimulinkFunction=on  FunctionName=bangBangControlAmp  FunctionVisibility=scoped  VariantControl=(inherit)
  How Much Muscle Model is Activated using Keyboard/Mouse : Constant  Value=0.0349
  y : ArgOut  DisableCoverage=on  ArgumentName=y
  wires:
  How Much Muscle Model is Activated using Keyboard/Mouse/1 -> y/1

== system InteractiveArmModel_R2021a_v1/Constants/betaE ==
  betaE : TriggerPort  TriggerType=function-call  IsSimulinkFunction=on  FunctionName=betaE  FunctionVisibility=scoped  VariantControl=(inherit)
  betaExtensor : Constant  Value=15
  y : ArgOut  DisableCoverage=on  ArgumentName=y
  wires:
  betaExtensor/1 -> y/1

== system InteractiveArmModel_R2021a_v1/Constants/betaF ==
  betaF : TriggerPort  TriggerType=function-call  IsSimulinkFunction=on  FunctionName=betaF  FunctionVisibility=scoped  VariantControl=(inherit)
  betaFlexor : Constant  Value=15
  y : ArgOut  DisableCoverage=on  ArgumentName=y
  wires:
  betaFlexor/1 -> y/1

== system InteractiveArmModel_R2021a_v1/Constants/errorThresh ==
  errorThresh : TriggerPort  TriggerType=function-call  IsSimulinkFunction=on  FunctionName=errorThresh  FunctionVisibility=scoped  VariantControl=(inherit)
  Error Threshold (rad) : Constant  Value=0.0349
  y : ArgOut  DisableCoverage=on  ArgumentName=y
  wires:
  Error Threshold (rad)/1 -> y/1

== system InteractiveArmModel_R2021a_v1/Constants/insertLoc ==
  insertLoc : TriggerPort  TriggerType=function-call  IsSimulinkFunction=on  FunctionName=insertLoc  FunctionVisibility=scoped  VariantControl=(inherit)
  Insertion Location : Constant  Value=0.1
  y : ArgOut  DisableCoverage=on  ArgumentName=y
  wires:
  Insertion Location/1 -> y/1

== system InteractiveArmModel_R2021a_v1/Constants/musNoise ==
  musNoise : TriggerPort  TriggerType=function-call  IsSimulinkFunction=on  FunctionName=musNoise  FunctionVisibility=scoped  VariantControl=(inherit)
  Mus Noise Constamt : Constant  Value=musNoise
  y : ArgOut  DisableCoverage=on  ArgumentName=y
  wires:
  Mus Noise Constamt/1 -> y/1

== system InteractiveArmModel_R2021a_v1/Constants/originLoc ==
  originLoc : TriggerPort  TriggerType=function-call  IsSimulinkFunction=on  FunctionName=originLoc  FunctionVisibility=scoped  VariantControl=(inherit)
  Origin Location : Constant  Value=0.9
  y : ArgOut  DisableCoverage=on  ArgumentName=y
  wires:
  Origin Location/1 -> y/1

== system InteractiveArmModel_R2021a_v1/Constants/startLoc ==
  startLoc : TriggerPort  TriggerType=function-call  IsSimulinkFunction=on  FunctionName=startLoc  FunctionVisibility=scoped  VariantControl=(inherit)
  Start Location (rad) : Constant  Value=1.57
  y : ArgOut  DisableCoverage=on  ArgumentName=y
  wires:
  Start Location (rad)/1 -> y/1

== system InteractiveArmModel_R2021a_v1/Constants/targetLoc ==
  targetLoc : TriggerPort  TriggerType=function-call  IsSimulinkFunction=on  FunctionName=targetLoc  FunctionVisibility=scoped  VariantControl=(inherit)
  Target Location (rad) : Constant  Value=2.5
  y : ArgOut  DisableCoverage=on  ArgumentName=y
  wires:
  Target Location (rad)/1 -> y/1

== system InteractiveArmModel_R2021a_v1/Constants/velThresh ==
  velThresh : TriggerPort  TriggerType=function-call  IsSimulinkFunction=on  FunctionName=velThresh  FunctionVisibility=scoped  VariantControl=(inherit)
  Velocity Threshold (rad/s) : Constant  Value=0.5
  y : ArgOut  DisableCoverage=on  ArgumentName=y
  wires:
  Velocity Threshold (rad/s)/1 -> y/1

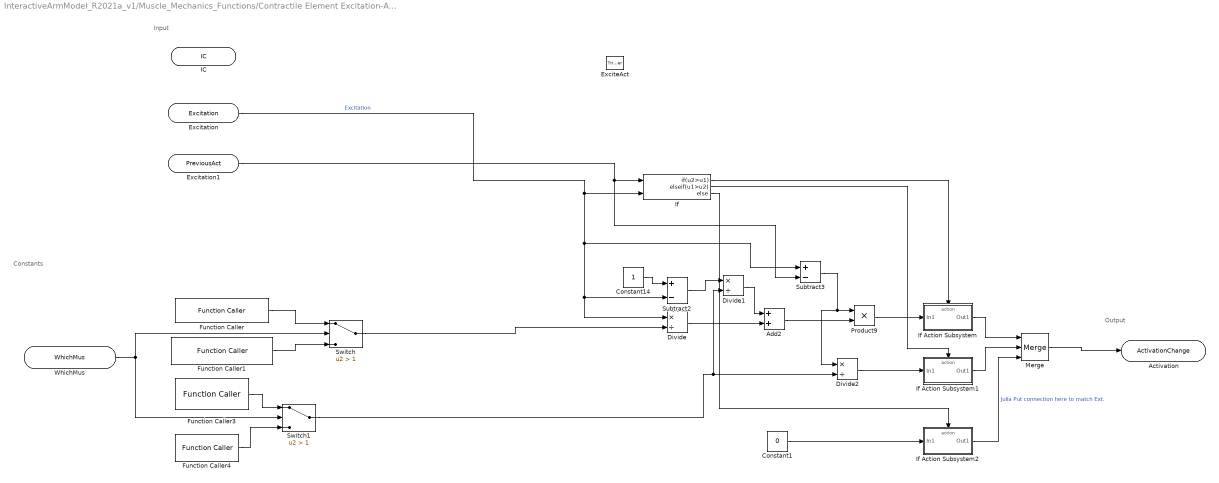
== system InteractiveArmModel_R2021a_v1/Muscle_Mechanics_Functions/Contractile Element Excitation-Activation Relation ==
  note: Output
  note: Input
  note: Constants
  ExciteAct : TriggerPort  TriggerType=function-call  IsSimulinkFunction=on  FunctionName=ExciteAct  FunctionVisibility=scoped  VariantControl=(inherit)
  Add2 : Sum
  Constant1 : Constant  Value=0  SampleTime=-1
  Constant14 : Constant  SampleTime=-1
  Divide : Product  Inputs=*/
  Divide1 : Product  Inputs=*/
  Divide2 : Product  Inputs=*/
  Function Caller : FunctionCaller  FunctionPrototype=y = Constants.CactF()  InputArgumentSpecifications=<Enter example>  OutputArgumentSpecifications=<Enter example>
  Function Caller1 : FunctionCaller  FunctionPrototype=y = Constants.CactE()  InputArgumentSpecifications=<Enter example>  OutputArgumentSpecifications=<Enter example>
  Function Caller3 : FunctionCaller  FunctionPrototype=y = Constants.CdeactF()  InputArgumentSpecifications=<Enter example>  OutputArgumentSpecifications=<Enter example>
  Function Caller4 : FunctionCaller  FunctionPrototype=y = Constants.CdeactE()  InputArgumentSpecifications=<Enter example>  OutputArgumentSpecifications=<Enter example>
  If : If  NumInputs=2  IfExpression=u2>u1  ElseIfExpressions=u1>u2
  If Action Subsystem : Subsystem  TreatAsAtomicUnit=on
  If Action Subsystem1 : Subsystem  TreatAsAtomicUnit=on
  If Action Subsystem2 : Subsystem  TreatAsAtomicUnit=on
  Merge : Merge  Inputs=3
  Product9 : Product
  Subtract2 : Sum  Inputs=+-
  Subtract3 : Sum  Inputs=+-
  Switch : Switch  Criteria=u2 > Threshold  Threshold=1
  Switch1 : Switch  Criteria=u2 > Threshold  Threshold=1
  IC : ArgIn  DisableCoverage=on  OutDataTypeStr=boolean  ArgumentName=IC
  Excitation : ArgIn  DisableCoverage=on  Port=2  ArgumentName=Excitation
  WhichMus : ArgIn  Port=3  ArgumentName=WhichMus
  Excitation1 : ArgIn  DisableCoverage=on  Port=4  ArgumentName=PreviousAct
  Activation : ArgOut  DisableCoverage=on  ArgumentName=ActivationChange
  wires:
  Function Caller/1 -> Switch/1
  Function Caller1/1 -> Switch/3
  Function Caller3/1 -> Switch1/1
  Function Caller4/1 -> Switch1/3
  WhichMus/1 -> Switch/2, Switch1/2
  Subtract3/1 -> Divide2/1, Product9/1
  If Action Subsystem2/1(Out1) -> Merge/3  "Julia Put connection here to match Ext."
  If/2 -> If Action Subsystem1/Action
  Constant1/1 -> If Action Subsystem2/1(In1)
  If/3 -> If Action Subsystem2/Action
  Divide/1 -> Add2/2
  Constant14/1 -> Subtract2/1
  Divide1/1 -> Add2/1
  Add2/1 -> Product9/2
  Switch1/1 -> Divide2/2, Divide1/2
  If Action Subsystem/1(Out1) -> Merge/1
  Divide2/1 -> If Action Subsystem1/1(In1)
  Subtract2/1 -> Divide1/1
  Switch/1 -> Divide/2
  If/1 -> If Action Subsystem/Action
  If Action Subsystem1/1(Out1) -> Merge/2
  Excitation/1 -> Divide/1, Subtract2/2, Subtract3/1, If/2  "Excitation"
  Product9/1 -> If Action Subsystem/1(In1)
  Excitation1/1 -> Subtract3/2, If/1
  Merge/1 -> Activation/1

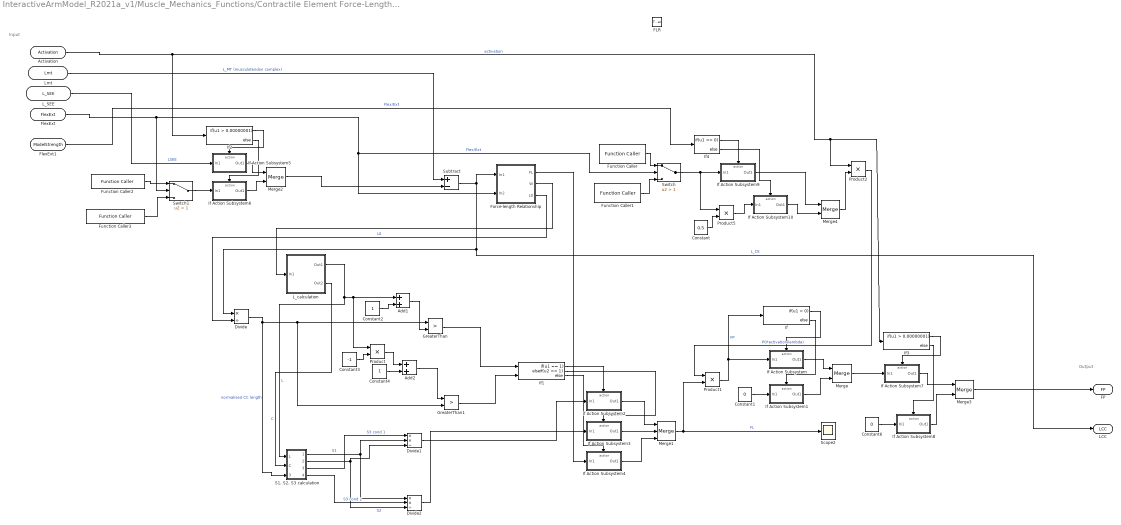
== system InteractiveArmModel_R2021a_v1/Muscle_Mechanics_Functions/Contractile Element Force-Length Relation ==
  note: Output
  note: Input
  FLR : TriggerPort  TriggerType=function-call  IsSimulinkFunction=on  FunctionName=FLR  FunctionVisibility=scoped  VariantControl=(inherit)
  Add1 : Sum
  Add2 : Sum
  Constant : Constant  Value=0.5
  Constant1 : Constant  Value=0
  Constant2 : Constant
  Constant3 : Constant  Value=-1
  Constant4 : Constant
  Constant6 : Constant  Value=0
  Divide : Product  Inputs=*/
  Divide1 : Product  Inputs=**/
  Divide2 : Product  Inputs=**/
  Force-length Relationship : Subsystem
  Function Caller : FunctionCaller  FunctionPrototype=y = Constants.P0F()  InputArgumentSpecifications=<Enter example>  OutputArgumentSpecifications=<Enter example>
  Function Caller1 : FunctionCaller  FunctionPrototype=y = Constants.P0E()  InputArgumentSpecifications=<Enter example>  OutputArgumentSpecifications=<Enter example>
  Function Caller2 : FunctionCaller  FunctionPrototype=y = Constants.Slack_lengthF()  InputArgumentSpecifications=<Enter example>  OutputArgumentSpecifications=<Enter example>
  Function Caller3 : FunctionCaller  FunctionPrototype=y = Constants.Slack_lengthE()  InputArgumentSpecifications=<Enter example>  OutputArgumentSpecifications=<Enter example>
  GreaterThan : RelationalOperator  Operator=>  OutDataTypeStr=boolean  RndMeth=Simplest
  GreaterThan1 : RelationalOperator  Operator=>  OutDataTypeStr=boolean  RndMeth=Simplest
  If : If
  If Action Subsystem : Subsystem  TreatAsAtomicUnit=on
  If Action Subsystem1 : Subsystem  TreatAsAtomicUnit=on
  If Action Subsystem10 : Subsystem  TreatAsAtomicUnit=on
  If Action Subsystem2 : Subsystem  TreatAsAtomicUnit=on
  If Action Subsystem3 : Subsystem  TreatAsAtomicUnit=on
  If Action Subsystem4 : Subsystem  TreatAsAtomicUnit=on
  If Action Subsystem5 : Subsystem  TreatAsAtomicUnit=on
  If Action Subsystem6 : Subsystem  TreatAsAtomicUnit=on
  If Action Subsystem7 : Subsystem  TreatAsAtomicUnit=on
  If Action Subsystem8 : Subsystem  TreatAsAtomicUnit=on
  If Action Subsystem9 : Subsystem  TreatAsAtomicUnit=on
  If1 : If  NumInputs=2  IfExpression=u1 == 1  ElseIfExpressions=u2 == 1
  If2 : If  IfExpression=u1 > 0.00000001
  If3 : If  IfExpression=u1 > 0.00000001
  If4 : If  IfExpression=u1 == 0
  L_calculation : Subsystem
  Merge{,2..4} (4 alike) : Merge
  Merge1 : Merge  Inputs=3
  Product{,1..2,5} (4 alike) : Product
  "S1, S2, S3 calculation" : Subsystem
  Scope2 : Scope
  Subtract : Sum  Inputs=+-
  Switch : Switch  Criteria=u2 > Threshold  Threshold=1
  Switch1 : Switch  Criteria=u2 > Threshold  Threshold=1
  Lmt : ArgIn  DisableCoverage=on  ArgumentName=Lmt
  L_SEE : ArgIn  DisableCoverage=on  Port=2  ArgumentName=L_SEE
  Activation : ArgIn  DisableCoverage=on  Port=3  ArgumentName=Activation
  FlexExt : ArgIn  DisableCoverage=on  Port=4  ArgumentName=FlexExt
  FlexExt1 : ArgIn  DisableCoverage=on  Port=5  ArgumentName=ModelStrength
  FP : ArgOut  DisableCoverage=on  ArgumentName=FP
  LCC : ArgOut  DisableCoverage=on  Port=2  ArgumentName=LCC
  wires:
  Force-length Relationship/3(L0) -> Divide/2  "L0"
  Product1/1 -> If Action Subsystem/1(In1), If/1  "FP"
  Product/1 -> Add2/1
  "S1, S2, S3 calculation"/1(Out1) -> Divide1/2, Divide2/1  "S1"
  "S1, S2, S3 calculation"/4(Out4) -> Divide2/2  "S3 cond 2"
  Force-length Relationship/2(W) -> L_calculation/1(In1)
  If1/2 -> If Action Subsystem3/Action
  "S1, S2, S3 calculation"/2(Out2) -> Divide1/3, Divide2/3  "S2"
  If1/1 -> If Action Subsystem2/Action
  Lmt/1 -> Subtract/1  "L_MT (musculotendon complex)"
  Add2/1 -> GreaterThan1/1
  Divide1/1 -> If Action Subsystem2/1(In1)
  If1/3 -> If Action Subsystem4/Action
  If Action Subsystem4/1(Out1) -> Merge1/3
  Add1/1 -> GreaterThan/2
  Constant3/1 -> Product/2
  If Action Subsystem3/1(Out1) -> Merge1/2
  If Action Subsystem2/1(Out1) -> Merge1/1
  "S1, S2, S3 calculation"/3(Out3) -> Divide1/1  "S3 cond 1"
  Merge1/1 -> Product1/2, Scope2/1  "FL"
  Divide/1 -> "S1, S2, S3 calculation"/3(normalised CC length), GreaterThan1/2, GreaterThan/1  "normalised CC length"
  Constant2/1 -> Add1/2
  Divide2/1 -> If Action Subsystem3/1(In1)
  L_calculation/2(Out2) -> "S1, S2, S3 calculation"/2(C)  "C"
  GreaterThan1/1 -> If1/2
  Force-length Relationship/1(FL) -> If Action Subsystem4/1(In1)
  L_calculation/1(Out1) -> Product/1, Add1/1, "S1, S2, S3 calculation"/1(L)  "L"
  GreaterThan/1 -> If1/1
  Product2/1 -> Product1/1  "P0*activation(lambda)"
  Constant4/1 -> Add2/2
  Subtract/1 -> LCC/1, Divide/1, Force-length Relationship/1(In1)  "L_CE"
  Activation/1 -> If2/1, Product2/1, If3/1  "activation"
  FlexExt/1 -> Switch1/2, Switch/2, Force-length Relationship/2(In2)  "Flex/Ext"
  Function Caller/1 -> Switch/1
  Function Caller1/1 -> Switch/3
  If/1 -> If Action Subsystem/Action
  If/2 -> If Action Subsystem1/Action
  Constant1/1 -> If Action Subsystem1/1(In1)
  If Action Subsystem/1(Out1) -> Merge/1
  If Action Subsystem1/1(Out1) -> Merge/2
  If2/1 -> If Action Subsystem5/Action
  If2/2 -> If Action Subsystem6/Action
  L_SEE/1 -> If Action Subsystem5/1(In1)  "LSEE"
  Switch1/1 -> If Action Subsystem6/1(In1)
  If Action Subsystem5/1(Out1) -> Merge2/1
  If Action Subsystem6/1(Out1) -> Merge2/2
  Merge2/1 -> Subtract/2
  Merge/1 -> If Action Subsystem7/1(In1)
  If3/1 -> If Action Subsystem7/Action
  If3/2 -> If Action Subsystem8/Action
  Constant6/1 -> If Action Subsystem8/1(In1)
  If Action Subsystem7/1(Out1) -> Merge3/1
  If Action Subsystem8/1(Out1) -> Merge3/2
  Merge3/1 -> FP/1
  Function Caller2/1 -> Switch1/1
  Function Caller3/1 -> Switch1/3
  Switch/1 -> Product5/1, If Action Subsystem9/1(In1)
  FlexExt1/1 -> If4/1  "Flex/Ext"
  If4/1 -> If Action Subsystem9/Action
  If Action Subsystem9/1(Out1) -> Merge4/1
  If4/2 -> If Action Subsystem10/Action
  If Action Subsystem10/1(Out1) -> Merge4/2
  Constant/1 -> Product5/2
  Product5/1 -> If Action Subsystem10/1(In1)
  Merge4/1 -> Product2/2
